simulink library "Lib_kinematics"  (R2024b)
settings: Solver=VariableStepAuto  StartTime=0.0  StopTime=10.0  RelTol=1e-3
undefined symbols (not defined in the file or in its folder): magnitude
settings Model: Creator=stefa  LastModifiedBy=stefa

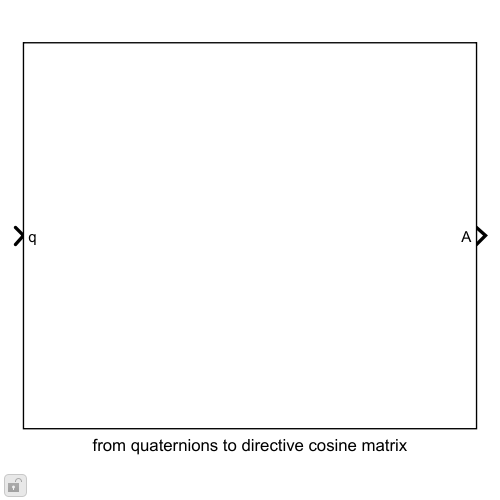
[thumbnail: Simulink's stored preview of the top-level diagram]
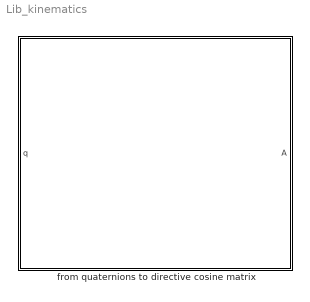
== system Lib_kinematics ==
  from quaternions to directive cosine matrix : Subsystem

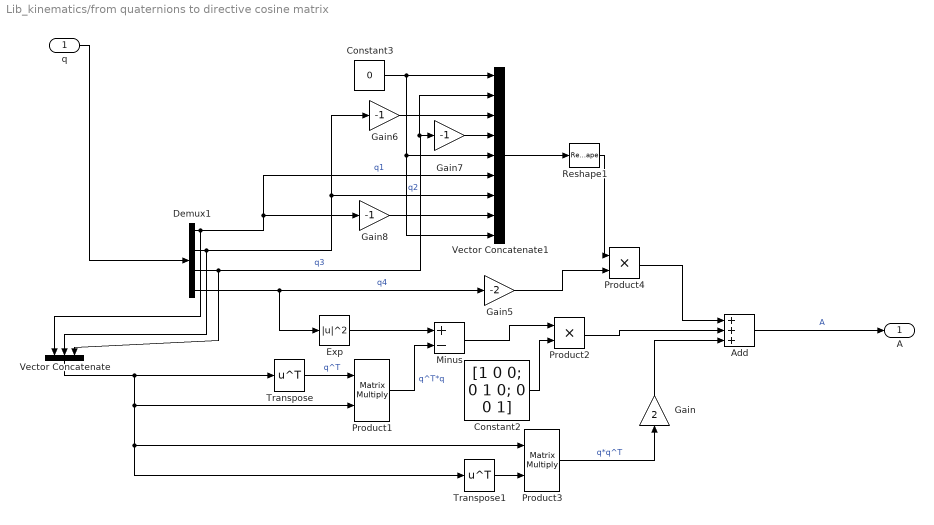
== system Lib_kinematics/from quaternions to directive cosine matrix ==
  q : Inport
  Add : Sum  Inputs=+++
  Constant2 : Constant  Value=[1 0 0; 0 1 0; 0 0 1]
  Constant3 : Constant  Value=0
  Demux1 : Demux
  Exp : Math  Operator=magnitude^2
  Gain : Gain  Gain=2
  Gain5 : Gain  Gain=-2
  Gain6 : Gain  Gain=-1
  Gain7 : Gain  Gain=-1
  Gain8 : Gain  Gain=-1
  Minus : Sum  Inputs=+-
  Product1 : Product  Multiplication=Matrix(*)
  Product2 : Product
  Product3 : Product  Multiplication=Matrix(*)
  Product4 : Product
  Reshape1 : Reshape  OutputDimensionality=Customize  OutputDimensions=[3,3]
  Transpose : Math  Operator=transpose
  Transpose1 : Math  Operator=transpose
  Vector Concatenate : Concatenate  NumInputs=3
  Vector Concatenate1 : Concatenate  NumInputs=9
  A : Outport
  wires:
  Demux1/4 -> Exp/1, Gain5/1  "q4"
  Vector Concatenate1/1 -> Reshape1/1
  Reshape1/1 -> Product4/1
  Constant3/1 -> Vector Concatenate1/9, Vector Concatenate1/5, Vector Concatenate1/1
  Gain7/1 -> Vector Concatenate1/4
  Demux1/2 -> Vector Concatenate1/7, Gain6/1, Vector Concatenate/2  "q2"
  Demux1/1 -> Vector Concatenate/1, Gain8/1, Vector Concatenate1/6  "q1"
  Transpose1/1 -> Product3/2
  Product1/1 -> Minus/2  "q^T*q"
  Exp/1 -> Minus/1
  Product2/1 -> Add/2
  q/1 -> Demux1/1
  Minus/1 -> Product2/1
  Product4/1 -> Add/1
  Add/1 -> A/1  "A"
  Product3/1 -> Gain/1  "q*q^T"
  Constant2/1 -> Product2/2
  Demux1/3 -> Vector Concatenate1/2, Gain7/1, Vector Concatenate/3  "q3"
  Transpose/1 -> Product1/1  "q^T"
  Gain6/1 -> Vector Concatenate1/3
  Gain8/1 -> Vector Concatenate1/8
  Gain5/1 -> Product4/2
  Vector Concatenate/1 -> Product3/1, Transpose1/1, Product1/2, Transpose/1
  Gain/1 -> Add/3
